simulink model "parameter_estimate"  (R2021a)
settings: Solver=VariableStepAuto  StartTime=0.0  StopTime=time_est  RelTol=1e-3
values from neighbouring files (symbols this model uses):
  Delta = block.DialogPrm(1).data    [battery_ekf.m]    (also in init_script_num.m = cur_est.Time(2)-cur_est.Time(1); num_diff_imp_valid.m = cur_est.Time(2)-cur_est.Time(1))
settings Model: Creator=saleh  LastModifiedBy=saleh

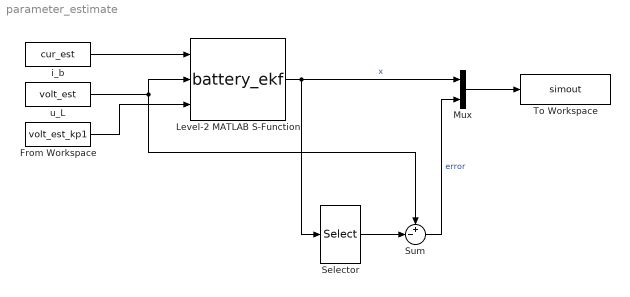
== system parameter_estimate ==
  From Workspace : FromWorkspace  VariableName=volt_est_kp1  SampleTime=Delta
  Level-2 MATLAB S-Function : M-S-Function  FunctionName=battery_ekf  Parameters=Delta, x0, P0, a, Z_k, W_k, Qe, Cg
  Mux : Mux  Inputs=2
  Selector : Selector  InputPortWidth=6  IndexOptions=Index vector (dialog)  Indices=6  OutputSizes=1
  Sum : Sum  Inputs=+-|
  To Workspace : ToWorkspace  VariableName=simout  SampleTime=-1
  i_b : FromWorkspace  VariableName=cur_est  SampleTime=Delta
  u_L : FromWorkspace  VariableName=volt_est  SampleTime=Delta
  wires:
  i_b/1 -> Level-2 MATLAB S-Function/1
  u_L/1 -> Sum/1, Level-2 MATLAB S-Function/2
  Level-2 MATLAB S-Function/1 -> Mux/1, Selector/1  "x"
  Selector/1 -> Sum/2
  Sum/1 -> Mux/2  "error"
  Mux/1 -> To Workspace/1
  From Workspace/1 -> Level-2 MATLAB S-Function/3
